simulink model "Demo_MultiUAV_ProQuek_Sep2013_1"  (Simulink 7.7)
settings: Solver=ode5  StartTime=0.0  StopTime=inf  FixedStep=sample_time  RelTol=1e-3
InitFcn:
  | sample_time=0.005;%0.004;%0.0025;%0.02;
  | sample_time_Vicon = 0.005;
  | DeltaT = 0.02;
  | g = 9.81;
  | H0 = g%0.3165;
  | Kl = 1;
  | 
  | Q6_mass = 0.73;
  | 
  | Q6_Omega_r = 1.5; %for horizon ref
  | Q6_Zeta_r = 0.5; %for horizon ref
  | Q6_Omega_r_h = 2;%for vertical ref
  | Q6_Zeta_r_h = 1; %for vertical ref
  | 
  | 
  | Q6_Omega = 1.5; %for horizon control
  | Q6_Zeta = 0.5; %for horizon control
  | Q6_Omega_h= 2; %for vertical control
  | Q6_Zeta_h = 0.7; %for vertical control
  | 
  | 
  | Q6_acc_max = 5;%horizontal max acc
  | Q6_acc_max_h = 3;%horizontal max acc
  | 
  | omega_circle = 72*pi/180;
  | omega_h = 0.1;%Ascending speed
  | PI = pi;
  | Circle_R = 2.5;
  | MAX_Height = -2;
libraries: X330_Control x26, simulink x17
(part 2 of 2)

== system Demo_MultiUAV_ProQuek_Sep2013_1/Vicon_Data/Raw Quad Pose from Vicon/Process Vicon Raw Data7/Flip_pi1 ==
  Angle : Inport
  Add : Sum  Inputs=-+
  Compare To Constant1 : simulink/Logic and Bit Operations/Compare To Constant  SystemSampleTime=-1  relop=>  const=pi  LogicOutDataTypeMode=uint8  ZeroCross=off
  Constant : Constant  Value=2*pi
  Data Type Duplicate : DataTypeDuplicate
  Flip_0_to_2pi : Subsystem
      mask Type: Flip zero to 2pi
      mask Description: Flips the inputs into the range zero to +2pi
      mask Help: Flips the inputs into the range zero to +2pi
      mask Display: disp('Flip_0_2pi')
  Switch : Switch  Criteria=u2 ~= 0
  Angle_Flip : Outport
  wires:
  Angle/1 -> Flip_0_to_2pi/1(Angle), Data Type Duplicate/2
  Flip_0_to_2pi/1(Angle_Flip) -> Switch/3, Compare To Constant1/1, Add/2
  Compare To Constant1/1 -> Switch/2
  Constant/1 -> Add/1
  Add/1 -> Switch/1
  Switch/1 -> Angle_Flip/1, Data Type Duplicate/1

== system Demo_MultiUAV_ProQuek_Sep2013_1/Vicon_Data/Raw Quad Pose from Vicon/Process Vicon Raw Data1/Flip_pi1/Flip_0_to_2pi ==
  Angle : Inport
  Add : Sum
  Compare To Constant1 : simulink/Logic and Bit Operations/Compare To Constant  SystemSampleTime=-1  relop=<  const=0  LogicOutDataTypeMode=uint8  ZeroCross=off
  Constant : Constant  Value=2*pi
  Data Type Duplicate : DataTypeDuplicate
  Flip_2pi : Subsystem
      mask Type: Flip -2pi to 2pi
      mask Description: Flips the inputs into the range -2pi to +2pi
      mask Help: Flips the inputs into the range -2pi to +2pi
      mask Display: disp('Flip_2pi')
  Switch : Switch  Criteria=u2 ~= 0
  Angle_Flip : Outport
  wires:
  Switch/1 -> Data Type Duplicate/1, Angle_Flip/1
  Angle/1 -> Data Type Duplicate/2, Flip_2pi/1(Angle)
  Add/1 -> Switch/1
  Constant/1 -> Add/1
  Compare To Constant1/1 -> Switch/2
  Flip_2pi/1(Angle_Flip) -> Switch/3, Add/2, Compare To Constant1/1

== system Demo_MultiUAV_ProQuek_Sep2013_1/Vicon_Data/Raw Quad Pose from Vicon/Process Vicon Raw Data2/Flip_pi1/Flip_0_to_2pi ==
  Angle : Inport
  Add : Sum
  Compare To Constant1 : simulink/Logic and Bit Operations/Compare To Constant  SystemSampleTime=-1  relop=<  const=0  LogicOutDataTypeMode=uint8  ZeroCross=off
  Constant : Constant  Value=2*pi
  Data Type Duplicate : DataTypeDuplicate
  Flip_2pi : Subsystem
      mask Type: Flip -2pi to 2pi
      mask Description: Flips the inputs into the range -2pi to +2pi
      mask Help: Flips the inputs into the range -2pi to +2pi
      mask Display: disp('Flip_2pi')
  Switch : Switch  Criteria=u2 ~= 0
  Angle_Flip : Outport
  wires:
  Flip_2pi/1(Angle_Flip) -> Compare To Constant1/1, Add/2, Switch/3
  Compare To Constant1/1 -> Switch/2
  Constant/1 -> Add/1
  Add/1 -> Switch/1
  Angle/1 -> Flip_2pi/1(Angle), Data Type Duplicate/2
  Switch/1 -> Angle_Flip/1, Data Type Duplicate/1

== system Demo_MultiUAV_ProQuek_Sep2013_1/Vicon_Data/Raw Quad Pose from Vicon/Process Vicon Raw Data3/Flip_pi1/Flip_0_to_2pi ==
  Angle : Inport
  Add : Sum
  Compare To Constant1 : simulink/Logic and Bit Operations/Compare To Constant  SystemSampleTime=-1  relop=<  const=0  LogicOutDataTypeMode=uint8  ZeroCross=off
  Constant : Constant  Value=2*pi
  Data Type Duplicate : DataTypeDuplicate
  Flip_2pi : Subsystem
      mask Type: Flip -2pi to 2pi
      mask Description: Flips the inputs into the range -2pi to +2pi
      mask Help: Flips the inputs into the range -2pi to +2pi
      mask Display: disp('Flip_2pi')
  Switch : Switch  Criteria=u2 ~= 0
  Angle_Flip : Outport
  wires:
  Flip_2pi/1(Angle_Flip) -> Compare To Constant1/1, Add/2, Switch/3
  Compare To Constant1/1 -> Switch/2
  Constant/1 -> Add/1
  Add/1 -> Switch/1
  Angle/1 -> Flip_2pi/1(Angle), Data Type Duplicate/2
  Switch/1 -> Angle_Flip/1, Data Type Duplicate/1

== system Demo_MultiUAV_ProQuek_Sep2013_1/Vicon_Data/Raw Quad Pose from Vicon/Process Vicon Raw Data4/Flip_pi1/Flip_0_to_2pi ==
  Angle : Inport
  Add : Sum
  Compare To Constant1 : simulink/Logic and Bit Operations/Compare To Constant  SystemSampleTime=-1  relop=<  const=0  LogicOutDataTypeMode=uint8  ZeroCross=off
  Constant : Constant  Value=2*pi
  Data Type Duplicate : DataTypeDuplicate
  Flip_2pi : Subsystem
      mask Type: Flip -2pi to 2pi
      mask Description: Flips the inputs into the range -2pi to +2pi
      mask Help: Flips the inputs into the range -2pi to +2pi
      mask Display: disp('Flip_2pi')
  Switch : Switch  Criteria=u2 ~= 0
  Angle_Flip : Outport
  wires:
  Switch/1 -> Data Type Duplicate/1, Angle_Flip/1
  Angle/1 -> Data Type Duplicate/2, Flip_2pi/1(Angle)
  Add/1 -> Switch/1
  Constant/1 -> Add/1
  Compare To Constant1/1 -> Switch/2
  Flip_2pi/1(Angle_Flip) -> Switch/3, Add/2, Compare To Constant1/1

== system Demo_MultiUAV_ProQuek_Sep2013_1/Vicon_Data/Raw Quad Pose from Vicon/Process Vicon Raw Data6/Flip_pi1/Flip_0_to_2pi ==
  Angle : Inport
  Add : Sum
  Compare To Constant1 : simulink/Logic and Bit Operations/Compare To Constant  SystemSampleTime=-1  relop=<  const=0  LogicOutDataTypeMode=uint8  ZeroCross=off
  Constant : Constant  Value=2*pi
  Data Type Duplicate : DataTypeDuplicate
  Flip_2pi : Subsystem
      mask Type: Flip -2pi to 2pi
      mask Description: Flips the inputs into the range -2pi to +2pi
      mask Help: Flips the inputs into the range -2pi to +2pi
      mask Display: disp('Flip_2pi')
  Switch : Switch  Criteria=u2 ~= 0
  Angle_Flip : Outport
  wires:
  Switch/1 -> Data Type Duplicate/1, Angle_Flip/1
  Angle/1 -> Data Type Duplicate/2, Flip_2pi/1(Angle)
  Add/1 -> Switch/1
  Constant/1 -> Add/1
  Compare To Constant1/1 -> Switch/2
  Flip_2pi/1(Angle_Flip) -> Switch/3, Add/2, Compare To Constant1/1

== system Demo_MultiUAV_ProQuek_Sep2013_1/Vicon_Data/Raw Quad Pose from Vicon/Process Vicon Raw Data7/Flip_pi1/Flip_0_to_2pi ==
  Angle : Inport
  Add : Sum
  Compare To Constant1 : simulink/Logic and Bit Operations/Compare To Constant  SystemSampleTime=-1  relop=<  const=0  LogicOutDataTypeMode=uint8  ZeroCross=off
  Constant : Constant  Value=2*pi
  Data Type Duplicate : DataTypeDuplicate
  Flip_2pi : Subsystem
      mask Type: Flip -2pi to 2pi
      mask Description: Flips the inputs into the range -2pi to +2pi
      mask Help: Flips the inputs into the range -2pi to +2pi
      mask Display: disp('Flip_2pi')
  Switch : Switch  Criteria=u2 ~= 0
  Angle_Flip : Outport
  wires:
  Flip_2pi/1(Angle_Flip) -> Compare To Constant1/1, Add/2, Switch/3
  Compare To Constant1/1 -> Switch/2
  Constant/1 -> Add/1
  Add/1 -> Switch/1
  Angle/1 -> Flip_2pi/1(Angle), Data Type Duplicate/2
  Switch/1 -> Angle_Flip/1, Data Type Duplicate/1

== system Demo_MultiUAV_ProQuek_Sep2013_1/Vicon_Data/Raw Quad Pose from Vicon/Process Vicon Raw Data1/Flip_pi1/Flip_0_to_2pi/Flip_2pi ==
  Angle : Inport
  Bias : Bias  Bias=-2*pi
  Constant : Constant  Value=2*pi
  Data Type Duplicate : DataTypeDuplicate
  Modulo : Math  Operator=mod  SaturateOnIntegerOverflow=on
  Sign1 : Signum
  Switch : Switch
  Angle_Flip : Outport
  wires:
  Switch/1 -> Data Type Duplicate/2, Angle_Flip/1
  Bias/1 -> Switch/3
  Sign1/1 -> Switch/2
  Modulo/1 -> Switch/1, Bias/1
  Constant/1 -> Modulo/2
  Angle/1 -> Data Type Duplicate/1, Sign1/1, Modulo/1

== system Demo_MultiUAV_ProQuek_Sep2013_1/Vicon_Data/Raw Quad Pose from Vicon/Process Vicon Raw Data2/Flip_pi1/Flip_0_to_2pi/Flip_2pi ==
  Angle : Inport
  Bias : Bias  Bias=-2*pi
  Constant : Constant  Value=2*pi
  Data Type Duplicate : DataTypeDuplicate
  Modulo : Math  Operator=mod  SaturateOnIntegerOverflow=on
  Sign1 : Signum
  Switch : Switch
  Angle_Flip : Outport
  wires:
  Angle/1 -> Modulo/1, Sign1/1, Data Type Duplicate/1
  Constant/1 -> Modulo/2
  Modulo/1 -> Bias/1, Switch/1
  Sign1/1 -> Switch/2
  Bias/1 -> Switch/3
  Switch/1 -> Angle_Flip/1, Data Type Duplicate/2

== system Demo_MultiUAV_ProQuek_Sep2013_1/Vicon_Data/Raw Quad Pose from Vicon/Process Vicon Raw Data3/Flip_pi1/Flip_0_to_2pi/Flip_2pi ==
  Angle : Inport
  Bias : Bias  Bias=-2*pi
  Constant : Constant  Value=2*pi
  Data Type Duplicate : DataTypeDuplicate
  Modulo : Math  Operator=mod  SaturateOnIntegerOverflow=on
  Sign1 : Signum
  Switch : Switch
  Angle_Flip : Outport
  wires:
  Angle/1 -> Modulo/1, Sign1/1, Data Type Duplicate/1
  Constant/1 -> Modulo/2
  Modulo/1 -> Bias/1, Switch/1
  Sign1/1 -> Switch/2
  Bias/1 -> Switch/3
  Switch/1 -> Angle_Flip/1, Data Type Duplicate/2

== system Demo_MultiUAV_ProQuek_Sep2013_1/Vicon_Data/Raw Quad Pose from Vicon/Process Vicon Raw Data4/Flip_pi1/Flip_0_to_2pi/Flip_2pi ==
  Angle : Inport
  Bias : Bias  Bias=-2*pi
  Constant : Constant  Value=2*pi
  Data Type Duplicate : DataTypeDuplicate
  Modulo : Math  Operator=mod  SaturateOnIntegerOverflow=on
  Sign1 : Signum
  Switch : Switch
  Angle_Flip : Outport
  wires:
  Switch/1 -> Data Type Duplicate/2, Angle_Flip/1
  Bias/1 -> Switch/3
  Sign1/1 -> Switch/2
  Modulo/1 -> Switch/1, Bias/1
  Constant/1 -> Modulo/2
  Angle/1 -> Data Type Duplicate/1, Sign1/1, Modulo/1

== system Demo_MultiUAV_ProQuek_Sep2013_1/Vicon_Data/Raw Quad Pose from Vicon/Process Vicon Raw Data6/Flip_pi1/Flip_0_to_2pi/Flip_2pi ==
  Angle : Inport
  Bias : Bias  Bias=-2*pi
  Constant : Constant  Value=2*pi
  Data Type Duplicate : DataTypeDuplicate
  Modulo : Math  Operator=mod  SaturateOnIntegerOverflow=on
  Sign1 : Signum
  Switch : Switch
  Angle_Flip : Outport
  wires:
  Switch/1 -> Data Type Duplicate/2, Angle_Flip/1
  Bias/1 -> Switch/3
  Sign1/1 -> Switch/2
  Modulo/1 -> Switch/1, Bias/1
  Constant/1 -> Modulo/2
  Angle/1 -> Data Type Duplicate/1, Sign1/1, Modulo/1

== system Demo_MultiUAV_ProQuek_Sep2013_1/Vicon_Data/Raw Quad Pose from Vicon/Process Vicon Raw Data7/Flip_pi1/Flip_0_to_2pi/Flip_2pi ==
  Angle : Inport
  Bias : Bias  Bias=-2*pi
  Constant : Constant  Value=2*pi
  Data Type Duplicate : DataTypeDuplicate
  Modulo : Math  Operator=mod  SaturateOnIntegerOverflow=on
  Sign1 : Signum
  Switch : Switch
  Angle_Flip : Outport
  wires:
  Angle/1 -> Modulo/1, Sign1/1, Data Type Duplicate/1
  Constant/1 -> Modulo/2
  Modulo/1 -> Bias/1, Switch/1
  Sign1/1 -> Switch/2
  Bias/1 -> Switch/3
  Switch/1 -> Angle_Flip/1, Data Type Duplicate/2

== stateflow chart UAV 3/Trajectory Logic/UAV SF1 ==
  state Landing
    state Decsending
      en:PosDesired = Pos;
      du:PosDesired[2] = (0 - PosDesired[2])*1*DeltaT + PosDesired[2] ;
    state CutThrottle
      du:HoverThrottle = (0.01 - HoverThrottle)*2*DeltaT + HoverThrottle ;
    (default) -> Decsending
    Decsending -> CutThrottle : [Pos[2] > -0.15]
  state Airborne
    state TakeOff
      du:HoverThrottle = (H0 - HoverThrottle)*2*DeltaT + HoverThrottle ;
    state Hover
      en: PosDesired[2] = -1;
    state Trajectory
      state SpiralAscend
        du: PosDesired[0] = Circle_R*sin(0.0 + T_circle*omega_circle);
        PosDesired[1] = Circle_R*cos(0.0 + T_circle*omega_circle);
        PosDesired[2] =max( MAX_Height ,-1 - T_circle*omega_h);
        T_circle = T_circle + DeltaT;
      state Circle2D
        du: PosDesired[0] = Circle_R*sin(90*PI/180 + T_circle*omega_circle);
        PosDesired[1] = Circle_R*cos(90*PI/180 + T_circle*omega_circle);
        T_circle = T_circle + DeltaT;
      state SpiralDescend
        du: PosDesired[0] = Circle_R*sin((720- 240/2)*PI/180 + T_circle*omega_circle);
        PosDesired[1] = Circle_R*cos((720- 240/2)*PI/180 + T_circle*omega_circle);
        PosDesired[2] =min(-1,MAX_Height  + T_circle*omega_h);
        T_circle = T_circle + DeltaT;
      state Hex1
        en: PosDesired[0] = 1.5*sin(90*PI/180);
        PosDesired[1] = 1.5*cos(90*PI/180);
        PosDesired[2] = -1;
      state Line2
        en: PosDesired[0] = -1; PosDesired[1] = 0.5; PosDesired[2] = -1;
      state Line1
        en: PosDesired[0] = 0; PosDesired[1] = 0.5; PosDesired[2] = -1;
      state Line3
        en: PosDesired[0] = 1; PosDesired[1] = 0.5; PosDesired[2] = -1;
      state Hex
        en: PosDesired[0] = 1.5*sin(90*PI/180); PosDesired[1] = 1.5*cos(90*PI/180);
      state Line4
        en: PosDesired[0] = 0; PosDesired[1] = 0.5; PosDesired[2] = -1;
      Circle2D -> SpiralAscend : [T_circle*omega_circle*180/PI > (390 +240)]
          | {T_circle =0.0;}
      SpiralAscend -> SpiralDescend : [T_circle*omega_circle *180/PI > (720-240/2)]
          | {T_circle =0.0;}
      SpiralDescend -> Hex1 : [T_circle*omega_circle *180/PI > (720-240/2)]
          | {T_circle =0.0;}
      (default) -> Line1 : {line_count = -1;}
      Line1 -> Line2 : after (10, sec)
      Line2 -> Line3 : after (5, sec)
      Line3 -> Line4 : after (5, sec)
      Hex -> Circle2D : after (10, sec)
          | {T_circle = 0.0;}
      Line4 -> Hex : after (5, sec)
    (default) -> TakeOff : {PosDesired = Pos;  PosDesired[2] = -1;}
    TakeOff -> Hover : after(5,sec)
        | {PosDesired = Pos;}
    Hover -> Trajectory : [RC[5] > 0]
    Trajectory -> Hover : [RC[5] < 0]
        | {PosDesired = Pos;}
  (default) -> Landing : {HoverThrottle=0.01;}
  Airborne -> Landing : [RC[6] < -0.5]
  Landing -> Airborne : [RC[6] > 0.5]
  data: PosDesired output double size=4; HoverThrottle output double size=1; Mode output uint8 size=3; RC input double size=8; Pos input double size=4; PerchPos input double size=4; DeltaT parameter double size=1; H0 parameter double size=1; Kl parameter double size=1; VelCmd local double size=2 =0; line_count local int8 size=1 =0; triangle_count local int8 size=1 =0; T_circle local double size=1; omega_circle parameter double size=1; PI parameter double size=1; omega_h parameter double size=1; Circle_R parameter double size=1; MAX_Height parameter double size=1

== stateflow chart UAV 4/Trajectory Logic/UAV SF1 ==
  state Landing
    state Decsending
      en:PosDesired = Pos;
      du:PosDesired[2] = (0 - PosDesired[2])*1*DeltaT + PosDesired[2] ;
    state CutThrottle
      du:HoverThrottle = (0.01 - HoverThrottle)*2*DeltaT + HoverThrottle ;
    (default) -> Decsending
    Decsending -> CutThrottle : [Pos[2] > -0.15]
  state Airborne
    state TakeOff
      du:HoverThrottle = (H0 - HoverThrottle)*2*DeltaT + HoverThrottle ;
    state Hover
      en: PosDesired[2] = -1;
    state Trajectory
      state SpiralAscend
        du: PosDesired[0] = Circle_R*sin(0.0 + T_circle*omega_circle);
        PosDesired[1] = Circle_R*cos(0.0 + T_circle*omega_circle);
        PosDesired[2] = max(MAX_Height ,-1 - T_circle*omega_h);
        T_circle = T_circle + DeltaT;
      state Circle2D
        du: PosDesired[0] = Circle_R*sin(270*PI/180 + T_circle*omega_circle);
        PosDesired[1] = Circle_R*cos(270*PI/180 + T_circle*omega_circle);
        T_circle = T_circle + DeltaT;
      state SpiralDescend
        du: PosDesired[0] = Circle_R*sin((720- 60/2)*PI/180 + T_circle*omega_circle);
        PosDesired[1] = Circle_R*cos((720- 60/2)*PI/180 + T_circle*omega_circle);
        PosDesired[2] =min(-1,MAX_Height  + T_circle*omega_h);
        T_circle = T_circle + DeltaT;
      state Hex1
        en: PosDesired[0] = 1.5*sin(270*PI/180);
        PosDesired[1] = 1.5*cos(270*PI/180);
        PosDesired[2] = -1;
      state Line2
        en: PosDesired[0] = -1; PosDesired[1] =-0.5; PosDesired[2] = -1;
      state Line1
        en: PosDesired[0] = 0; PosDesired[1] = -0.5; PosDesired[2] = -1;
      state Line3
        en: PosDesired[0] = 1; PosDesired[1] =-0.5; PosDesired[2] = -1;
      state Hex
        en: PosDesired[0] = 1.5*sin(270*PI/180); PosDesired[1] = 1.5*cos(270*PI/180);
      state Line4
        en: PosDesired[0] = 0; PosDesired[1] = -0.5; PosDesired[2] = -1;
      Circle2D -> SpiralAscend : [T_circle*omega_circle*180/PI > (390 +60)]
          | {T_circle =0.0;}
      SpiralAscend -> SpiralDescend : [T_circle*omega_circle *180/PI > (720-60/2)]
          | {T_circle =0.0;}
      SpiralDescend -> Hex1 : [T_circle*omega_circle *180/PI > (720-60/2)]
          | {T_circle =0.0;}
      (default) -> Line1 : {line_count = -1;}
      Line1 -> Line2 : after (10, sec)
      Line2 -> Line3 : after (5, sec)
      Line3 -> Line4 : after (5, sec)
      Hex -> Circle2D : after (10, sec)
          | {T_circle = 0.0;}
      Line4 -> Hex : after (5, sec)
    (default) -> TakeOff : {PosDesired = Pos;  PosDesired[2] = -1;}
    TakeOff -> Hover : after(5,sec)
        | {PosDesired = Pos;}
    Hover -> Trajectory : [RC[5] > 0]
    Trajectory -> Hover : [RC[5] < 0]
        | {PosDesired = Pos;}
  (default) -> Landing : {HoverThrottle=0.01;}
  Airborne -> Landing : [RC[6] < -0.5]
  Landing -> Airborne : [RC[6] > 0.5]
  data: PosDesired output double size=4; HoverThrottle output double size=1; Mode output uint8 size=3; RC input double size=8; Pos input double size=4; PerchPos input double size=4; DeltaT parameter double size=1; H0 parameter double size=1; Kl parameter double size=1; VelCmd local double size=2 =0; line_count local int8 size=1 =0; triangle_count local int8 size=1 =0; T_circle local double size=1; omega_circle parameter double size=1; PI parameter double size=1; omega_h parameter double size=1; Circle_R parameter double size=1; MAX_Height parameter double size=1

== stateflow chart UAV 5/Trajectory Logic/UAV SF1 ==
  state Landing
    state Decsending
      en:PosDesired = Pos;
      du:PosDesired[2] = (0 - PosDesired[2])*1*DeltaT + PosDesired[2] ;
    state CutThrottle
      du:HoverThrottle = (0.01 - HoverThrottle)*2*DeltaT + HoverThrottle ;
    (default) -> Decsending
    Decsending -> CutThrottle : [Pos[2] > -0.15]
  state Airborne
    state TakeOff
      du:HoverThrottle = (H0 - HoverThrottle)*2*DeltaT + HoverThrottle ;
    state Hover
      en: PosDesired[2] = -1;
    state Trajectory
      state SpiralAscend
        du: PosDesired[0] = Circle_R*sin(0.0 + T_circle*omega_circle);
        PosDesired[1] = Circle_R*cos(0.0 + T_circle*omega_circle);
        PosDesired[2] = max(MAX_Height ,-1 - T_circle*omega_h);
        T_circle = T_circle + DeltaT;
      state Circle2D
        du: PosDesired[0] = Circle_R*sin(150*PI/180 + T_circle*omega_circle);
        PosDesired[1] = Circle_R*cos(150*PI/180 + T_circle*omega_circle);
        T_circle = T_circle + DeltaT;
      state SpiralDescend
        du: PosDesired[0] = Circle_R*sin((720- 180/2)*PI/180 + T_circle*omega_circle);
        PosDesired[1] = Circle_R*cos((720- 180/2)*PI/180 + T_circle*omega_circle);
        PosDesired[2] =min(-1,MAX_Height  + T_circle*omega_h);
        T_circle = T_circle + DeltaT;
      state Hex1
        en: PosDesired[0] = 1.5*sin(150*PI/180);
        PosDesired[1] = 1.5*cos(150*PI/180);
        PosDesired[2] = -1;
      state Line2
        en: PosDesired[0] = -1; PosDesired[1] =-1.5; PosDesired[2] = -1;
      state Line1
        en: PosDesired[0] = 0; PosDesired[1] = -1.5; PosDesired[2] = -1;
      state Line3
        en: PosDesired[0] = 1; PosDesired[1] =-1.5; PosDesired[2] = -1;
      state Hex
        en: PosDesired[0] = 1.5*sin(150*PI/180); PosDesired[1] = 1.5*cos(150*PI/180);
      state Line4
        en: PosDesired[0] = 0; PosDesired[1] = -1.5; PosDesired[2] = -1;
      Circle2D -> SpiralAscend : [T_circle*omega_circle*180/PI > (390 +180)]
          | {T_circle =0.0;}
      SpiralAscend -> SpiralDescend : [T_circle*omega_circle *180/PI > (720-180/2)]
          | {T_circle =0.0;}
      SpiralDescend -> Hex1 : [T_circle*omega_circle *180/PI > (720-180/2)]
          | {T_circle =0.0;}
      (default) -> Line1 : {line_count = -1;}
      Line1 -> Line2 : after (10, sec)
      Line2 -> Line3 : after (5, sec)
      Line3 -> Line4 : after (5, sec)
      Hex -> Circle2D : after (10, sec)
          | {T_circle = 0.0;}
      Line4 -> Hex : after (5, sec)
    (default) -> TakeOff : {PosDesired = Pos;  PosDesired[2] = -1;}
    TakeOff -> Hover : after(5,sec)
        | {PosDesired = Pos;}
    Hover -> Trajectory : [RC[5] > 0]
    Trajectory -> Hover : [RC[5] < 0]
        | {PosDesired = Pos;}
  (default) -> Landing : {HoverThrottle=0.01;}
  Airborne -> Landing : [RC[6] < -0.5]
  Landing -> Airborne : [RC[6] > 0.5]
  data: PosDesired output double size=4; HoverThrottle output double size=1; Mode output uint8 size=3; RC input double size=8; Pos input double size=4; PerchPos input double size=4; DeltaT parameter double size=1; H0 parameter double size=1; Kl parameter double size=1; VelCmd local double size=2 =0; line_count local int8 size=1 =0; triangle_count local int8 size=1 =0; T_circle local double size=1; omega_circle parameter double size=1; PI parameter double size=1; omega_h parameter double size=1; Circle_R parameter double size=1; MAX_Height parameter double size=1

== stateflow chart UAV 1/Trajectory Logic/UAV SF1 ==
  state Landing
    state Decsending
      en:PosDesired = Pos;
      du:PosDesired[2] = (0 - PosDesired[2])*1*DeltaT + PosDesired[2] ;
    state CutThrottle
      du:HoverThrottle = (0.01 - HoverThrottle)*2*DeltaT + HoverThrottle ;
    (default) -> Decsending
    Decsending -> CutThrottle : [Pos[2] > -0.15]
  state Airborne
    state TakeOff
      du:HoverThrottle = (H0 - HoverThrottle)*2*DeltaT + HoverThrottle ;
    state Hover
      en: PosDesired[2] = -1;
    state Trajectory
      state SpiralDescend
        du: PosDesired[0] = Circle_R*sin( (720- 300/2)*PI/180 + T_circle*omega_circle);
        PosDesired[1] = Circle_R*cos((720- 300/2)*PI/180 + T_circle*omega_circle);
        PosDesired[2] =min(-1,MAX_Height  + T_circle*omega_h);
        T_circle = T_circle + DeltaT;
      state Hex1
        en: PosDesired[0] = 1.5*sin(30*PI/180);
        PosDesired[1] = 1.5*cos(30*PI/180);
        PosDesired[2] = -1;
      state SpiralAscend
        du: PosDesired[0] = Circle_R*sin(0.0 + T_circle*omega_circle);
        PosDesired[1] = Circle_R*cos(0.0 + T_circle*omega_circle);
        PosDesired[2] = max(MAX_Height ,-1 - T_circle*omega_h);
        T_circle = T_circle + DeltaT;
      state Circle2D
        du: PosDesired[0] = Circle_R*sin(30*PI/180 + T_circle*omega_circle);
        PosDesired[1] = Circle_R*cos(30*PI/180 + T_circle*omega_circle);
        T_circle = T_circle + DeltaT;
      state Line2
        en: PosDesired[0] = -1; PosDesired[1] = 2.5; PosDesired[2] = -1;
      state Line1
        en: PosDesired[0] = 0; PosDesired[1] = 2.5; PosDesired[2] = -1;
      state Line3
        en: PosDesired[0] = 1; PosDesired[1] = 2.5; PosDesired[2] = -1;
      state Hex
        en: PosDesired[0] = 1.5*sin(30*PI/180); PosDesired[1] = 1.5*cos(30*PI/180);
      state Line4
        en: PosDesired[0] = 0; PosDesired[1] = 2.5; PosDesired[2] = -1;
      SpiralDescend -> Hex1 : [T_circle*omega_circle *180/PI > (720- 300/2)]
          | {T_circle =0.0;}
      SpiralAscend -> SpiralDescend : [T_circle*omega_circle *180/PI > (720- 300/2)]
          | {T_circle =0.0;}
      Circle2D -> SpiralAscend : [T_circle*omega_circle*180/PI > (390 +300)]
          | {T_circle =0.0;}
      (default) -> Line1 : {line_count = -1;}
      Line1 -> Line2 : after (10, sec)
      Line2 -> Line3 : after (5, sec)
      Line3 -> Line4 : after (5, sec)
      Hex -> Circle2D : after (10, sec)
          | {T_circle = 0.0;}
      Line4 -> Hex : after (5, sec)
    (default) -> TakeOff : {PosDesired = Pos;  PosDesired[2] = -1;}
    TakeOff -> Hover : after(5,sec)
        | {PosDesired = Pos;}
    Hover -> Trajectory : [RC[5] > 0]
    Trajectory -> Hover : [RC[5] < 0]
        | {PosDesired = Pos;}
  (default) -> Landing : {HoverThrottle=0.01;}
  Airborne -> Landing : [RC[6] < -0.5]
  Landing -> Airborne : [RC[6] > 0.5]
  data: PosDesired output double size=4; HoverThrottle output double size=1; Mode output uint8 size=3; RC input double size=8; Pos input double size=4; PerchPos input double size=4; DeltaT parameter double size=1; H0 parameter double size=1; Kl parameter double size=1; VelCmd local double size=2 =0; line_count local int8 size=1 =0; triangle_count local int8 size=1 =0; T_circle local double size=1; omega_circle parameter double size=1; PI parameter double size=1; omega_h parameter double; Circle_R parameter double size=1; MAX_Height parameter double size=1

== stateflow chart UAV 6/Trajectory Logic/UAV SF ==
  state Landing
    state Decsending
      en:PosDesired = Pos;
      du:PosDesired[2] = (0 - PosDesired[2])*1*DeltaT + PosDesired[2] ;
    state CutThrottle
      du:HoverThrottle = (0.01 - HoverThrottle)*2*DeltaT + HoverThrottle ;
    (default) -> Decsending
    Decsending -> CutThrottle : [Pos[2] > -0.15]
  state Airborne
    state TakeOff
      du:HoverThrottle = (H0 - HoverThrottle)*2*DeltaT + HoverThrottle ;
    state Hover
      en: PosDesired[2] = -1;
    state Trajectory
      state SpiralAscend
        du: PosDesired[0] = Circle_R*sin(0.0 + T_circle*omega_circle);
        PosDesired[1] = Circle_R*cos(0.0 + T_circle*omega_circle);
        PosDesired[2] = max(MAX_Height ,-1 - T_circle*omega_h);
        T_circle = T_circle + DeltaT;
      state Circle2D
        du: PosDesired[0] = Circle_R*sin(210*PI/180 + T_circle*omega_circle);
        PosDesired[1] = Circle_R*cos(210*PI/180 + T_circle*omega_circle);
        T_circle = T_circle + DeltaT;
      state SpiralDescend
        du: PosDesired[0] = Circle_R*sin( (720-120/2)*PI/180 + T_circle*omega_circle);
        PosDesired[1] = Circle_R*cos((720-120/2)*PI/180 + T_circle*omega_circle);
        PosDesired[2] =min(-1,MAX_Height  + T_circle*omega_h);
        T_circle = T_circle + DeltaT;
      state Hex1
        en: PosDesired[0] = 1.5*sin(210*PI/180);
        PosDesired[1] = 1.5*cos(210*PI/180);
        PosDesired[2] = -1;
      state Line2
        en: PosDesired[0] = -1; PosDesired[1] = -2.5; PosDesired[2] = -1;
      state Line1
        en: PosDesired[0] = 0; PosDesired[1] = -2.5; PosDesired[2] = -1;
      state Line3
        en: PosDesired[0] = 1; PosDesired[1] = -2.5; PosDesired[2] = -1;
      state Hex
        en: PosDesired[0] = 1.5*sin(210*PI/180); PosDesired[1] = 1.5*cos(210*PI/180);
      state Line4
        en: PosDesired[0] = 0; PosDesired[1] = -2.5; PosDesired[2] = -1;
      Circle2D -> SpiralAscend : [T_circle*omega_circle*180/PI > (390 +120)]
          | {T_circle =0.0;}
      SpiralAscend -> SpiralDescend : [T_circle*omega_circle *180/PI > (720-120/2)]
          | {T_circle =0.0;}
      SpiralDescend -> Hex1 : [T_circle*omega_circle *180/PI > (720-120/2)]
          | {T_circle =0.0;}
      (default) -> Line1 : {line_count = -1;}
      Line1 -> Line2 : after (10, sec)
      Line2 -> Line3 : after (5, sec)
      Line3 -> Line4 : after (5, sec)
      Hex -> Circle2D : after (10, sec)
          | {T_circle = 0.0;}
      Line4 -> Hex : after (5, sec)
    (default) -> TakeOff : {PosDesired = Pos;  PosDesired[2] = -1;}
    TakeOff -> Hover : after(5,sec)
        | {PosDesired = Pos;}
    Hover -> Trajectory : [RC[5] > 0]
    Trajectory -> Hover : [RC[5] < 0]
        | {PosDesired = Pos;}
  (default) -> Landing : {HoverThrottle=0.01;}
  Airborne -> Landing : [RC[6] < -0.5]
  Landing -> Airborne : [RC[6] > 0.5]
  data: PosDesired output double size=4; HoverThrottle output double size=1; Mode output uint8 size=3; RC input double size=8; Pos input double size=4; PerchPos input double size=4; DeltaT parameter double size=1; H0 parameter double size=1; Kl parameter double size=1; VelCmd local double size=2 =0; line_count local int8 size=1 =0; triangle_count local int8 size=1 =0; T_circle local double size=1; omega_circle parameter double size=1; PI parameter double size=1; omega_h parameter double size=1; Circle_R parameter double size=1; MAX_Height parameter double size=1
